simulink model "dsPIC33CK256MP508_MCLV2_SMO"  (R2021b)
settings: Solver=FixedStepDiscrete  StartTime=0.0  StopTime=10  FixedStep=.00005  RelTol=1e-3  EnableMultiTasking=on
PreLoadFcn:
  | dsPIC33CK256MP508_MCLV2_SMO_data;
InitFcn:
  | dsPIC33CK256MP508_MCLV2_SMO_data;
undefined symbols (not defined in the file): AN1, B0, B2, C9, D6, DiscIntNeverNeededParam, inverter, MaxPer, mcb_isCodeGenVar, mcb_isSimVar, P32, P57, P70, PI_params, Pin, pmsm, PU_System, PWM1max, PWM_frequency, Resol, s, Speed_openLoop, Ts, Ts_speed, us
libraries: mcbcontrolslib x13, MCHP_Blockset x13, simulink x10, mcbplantlib x1, autolibpmsmexterior x1
(part 3 of 3)

== matlab function dsPIC33CK256MP508_MCLV2_SMO/Current Control/Input Scaling/Sliding Mode Observer/smo/AN1078 Saturation1 ==
  data: u input; y output
 function y = fcn(u)
 
max=0.005;kslide=1;

if  abs(u) <=max
    y=(u*kslide)/max;
      
elseif   u > 0
    y = kslide;
    
else    
    y=-kslide;
    
end
